simulink subsystem "CheckInput"  (R2021a)
settings: Solver=VariableStepAuto  StartTime=0.0  StopTime=10.0  RelTol=1e-3
undefined symbols (not defined in the file): ErrCodeIn, NoErr, RangeLwIn, RangeUpIn
libraries: simulink x1
settings Model: Creator=zurnmar  LastModifiedBy=zurnmar

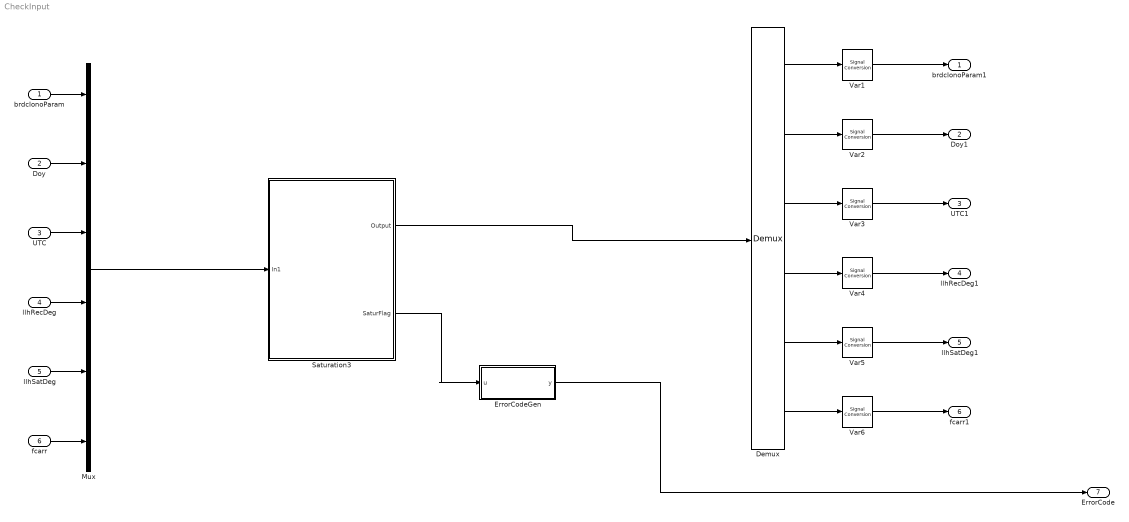
== system CheckInput ==
  brdcIonoParam : Inport
  Doy : Inport  Port=2
  UTC : Inport  Port=3
  llhRecDeg : Inport  Port=4
  llhSatDeg : Inport  Port=5
  fcarr : Inport  Port=6
  Demux : Demux  Outputs=6
  ErrorCodeGen : Subsystem
  Mux : Mux  Inputs=6
  Saturation3 : Subsystem
      settings: RTWFcnNameOpts=Use subsystem name
  Var{1..6} (6 alike) : SignalConversion  OverrideOpt=off
  brdcIonoParam1 : Outport
  Doy1 : Outport  Port=2
  UTC1 : Outport  Port=3
  llhRecDeg1 : Outport  Port=4
  llhSatDeg1 : Outport  Port=5
  fcarr1 : Outport  Port=6
  ErrorCode : Outport  Port=7
  wires:
  ErrorCodeGen/1(y) -> ErrorCode/1
  llhSatDeg/1 -> Mux/5
  llhRecDeg/1 -> Mux/4
  brdcIonoParam/1 -> Mux/1
  fcarr/1 -> Mux/6
  UTC/1 -> Mux/3
  Doy/1 -> Mux/2
  Mux/1 -> Saturation3/1(In1)
  Saturation3/1(Output) -> Demux/1
  Saturation3/2(SaturFlag) -> ErrorCodeGen/1(u)
  Demux/6 -> Var6/1
  Demux/5 -> Var5/1
  Demux/4 -> Var4/1
  Demux/3 -> Var3/1
  Demux/2 -> Var2/1
  Demux/1 -> Var1/1
  Var1/1 -> brdcIonoParam1/1
  Var2/1 -> Doy1/1
  Var3/1 -> UTC1/1
  Var4/1 -> llhRecDeg1/1
  Var5/1 -> llhSatDeg1/1
  Var6/1 -> fcarr1/1

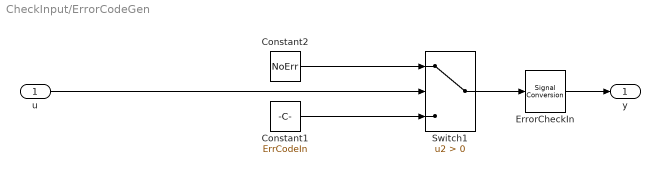
== system CheckInput/ErrorCodeGen ==
  u : Inport
  Constant1 : Constant  Value=ErrCodeIn  OutDataTypeStr=uint16
  Constant2 : Constant  Value=NoErr
  ErrorCheckIn : SignalConversion  OverrideOpt=off
  Switch1 : Switch  Criteria=u2 > Threshold
  y : Outport
  wires:
  ErrorCheckIn/1 -> y/1
  Switch1/1 -> ErrorCheckIn/1
  Constant1/1 -> Switch1/3
  Constant2/1 -> Switch1/1
  u/1 -> Switch1/2

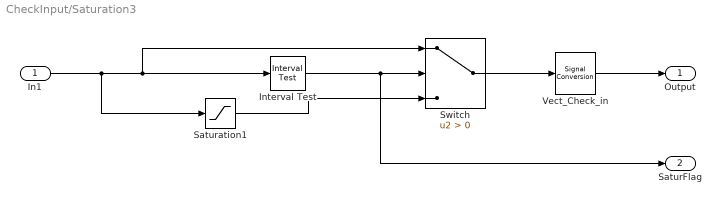
== system CheckInput/Saturation3 ==
  In1 : Inport
  Interval Test : simulink/Logic and Bit Operations/Interval Test  IntervalClosedRight=on  uplimit=RangeUpIn  IntervalClosedLeft=on  lowlimit=RangeLwIn  OutDataTypeStr=boolean
  Saturation1 : Saturate  UpperLimit=RangeUpIn  LowerLimit=RangeLwIn
  Switch : Switch  Criteria=u2 > Threshold
  Vect_Check_in : SignalConversion  OverrideOpt=off
  Output : Outport
  SaturFlag : Outport  Port=2
  wires:
  Interval Test/1 -> Switch/2, SaturFlag/1
  Vect_Check_in/1 -> Output/1
  Switch/1 -> Vect_Check_in/1
  In1/1 -> Saturation1/1, Interval Test/1, Switch/1
  Saturation1/1 -> Switch/3
